simulink model "test"  (Simulink 7.8)
settings: Solver=ode45  StartTime=0.0  StopTime=10.0  RelTol=1e-3
libraries: dsparch4 x3, commnoisgen2 x1
settings Model: Creator=deep  LastModifiedBy=deep

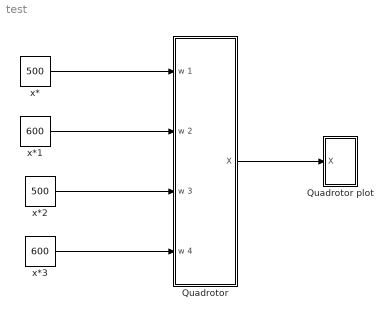
== system test ==
  Quadrotor : Subsystem  AncestorBlock=roblocks/Dynamics/Quadrotor
  Quadrotor plot : Subsystem  AncestorBlock=roblocks/Robot Graphics/Quadrotor plot
  x* : Constant  Value=500
  x*1 : Constant  Value=600
  x*2 : Constant  Value=500
  x*3 : Constant  Value=600
  wires:
  x*/1 -> Quadrotor/1(w 1)
  x*1/1 -> Quadrotor/2(w 2)
  x*2/1 -> Quadrotor/3(w 3)
  x*3/1 -> Quadrotor/4(w 4)
  Quadrotor/1(X) -> Quadrotor plot/1(X)

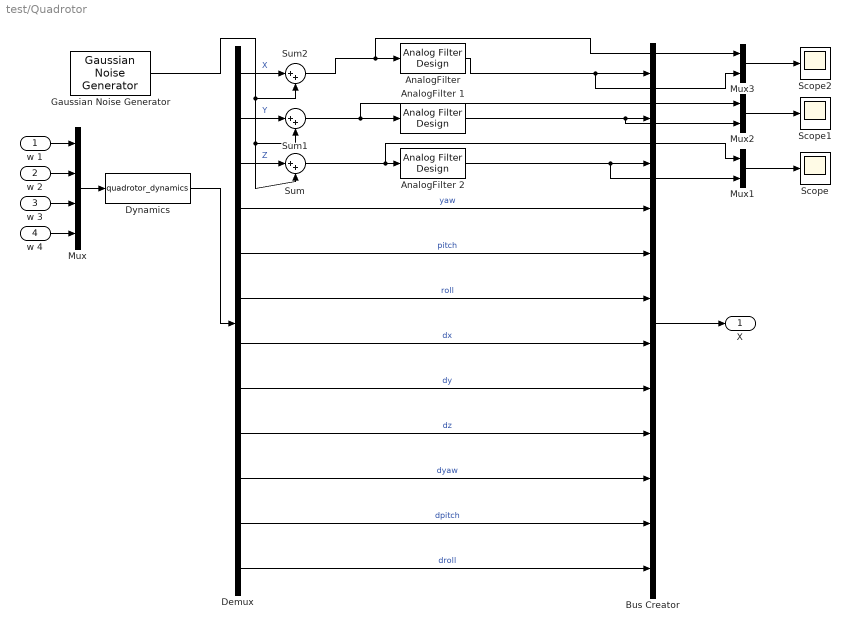
== system test/Quadrotor ==
  w 1 : Inport
  w 2 : Inport  Port=2
  w 3 : Inport  Port=3
  w 4 : Inport  Port=4
  "AnalogFilter " : dsparch4/Analog Filter Design  method=Butterworth  filttype=Lowpass  N=8  Wlo=10  Whi=80  Rp=2  Rs=40
  "AnalogFilter 1 " : dsparch4/Analog Filter Design  method=Butterworth  filttype=Lowpass  N=8  Wlo=10  Whi=80  Rp=2  Rs=40
  AnalogFilter 2 : dsparch4/Analog Filter Design  method=Butterworth  filttype=Lowpass  N=8  Wlo=10  Whi=80  Rp=2  Rs=40
  Bus Creator : BusCreator  Inputs=12
  Demux : Demux  Outputs=12
  Dynamics : S-Function  FunctionName=quadrotor_dynamics  Parameters=quad  EnableBusSupport=off
  Gaussian Noise Generator : commnoisgen2/Gaussian Noise Generator  m=0  d=0  s=0  Ts=0.01  frameBased=off  sampPerFrame=1  orient=off  outDataType=double
  Mux : Mux
  Mux1 : Mux  Inputs=2
  Mux2 : Mux  Inputs=2
  Mux3 : Mux  Inputs=2
  Scope : Scope
  Scope1 : Scope
      settings: SaveName=ScopeData13
  Scope2 : Scope
      settings: YMin=1.7  YMax=2.4  SaveName=ScopeData14
  Sum : Sum  Inputs=|++
  Sum1 : Sum  Inputs=|++
  Sum2 : Sum  Inputs=|++
  X : Outport
  wires:
  Mux/1 -> Dynamics/1
  Demux/4 -> Bus Creator/4  "yaw"
  Demux/5 -> Bus Creator/5  "pitch"
  w 1/1 -> Mux/1
  w 2/1 -> Mux/2
  w 3/1 -> Mux/3
  w 4/1 -> Mux/4
  Demux/7 -> Bus Creator/7  "dx"
  Demux/9 -> Bus Creator/9  "dz"
  Demux/6 -> Bus Creator/6  "roll"
  Demux/8 -> Bus Creator/8  "dy"
  Bus Creator/1 -> X/1
  Dynamics/1 -> Demux/1
  Demux/10 -> Bus Creator/10  "dyaw"
  Demux/11 -> Bus Creator/11  "dpitch"
  Demux/12 -> Bus Creator/12  "droll"
  Demux/3 -> Sum/1  "Z"
  Gaussian Noise Generator/1 -> Sum/2, Sum1/2, Sum2/2
  Sum/1 -> AnalogFilter 2/1, Mux1/1
  Mux1/1 -> Scope/1
  AnalogFilter 2/1 -> Bus Creator/3, Mux1/2
  Demux/2 -> Sum1/1  "Y"
  Sum1/1 -> "AnalogFilter 1 "/1, Mux2/1
  "AnalogFilter 1 "/1 -> Mux2/2, Bus Creator/2
  Demux/1 -> Sum2/1  "X"
  Sum2/1 -> "AnalogFilter "/1, Mux3/1
  "AnalogFilter "/1 -> Bus Creator/1, Mux3/2
  Mux3/1 -> Scope2/1
  Mux2/1 -> Scope1/1

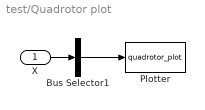
== system test/Quadrotor plot ==
  X : Inport
  Bus Selector1 : BusSelector  OutputSignals=signal1,signal2,signal3,yaw,pitch,roll  OutputAsBus=on
  Plotter : S-Function  FunctionName=quadrotor_plot  Parameters=[2,10], 1, 1  EnableBusSupport=off
  wires:
  X/1 -> Bus Selector1/1
  Bus Selector1/1 -> Plotter/1
